simulink library "tetherInternalForces_ul"  (R2018b)
settings: Solver=VariableStepAuto  StartTime=0.0  StopTime=10.0  RelTol=1e-3
values from neighbouring files (symbols this model uses):
  dia_t = 0.01    [tetherInternalForces_ts.m]
  E = 3.8e9    (= 3800000000)    [tetherInternalForces_ts.m]
  mass = 100    [tetherInternalForces_ts.m]
  N = 4    [tetherInternalForces_ts.m]
  zeta = 0.05    [tetherInternalForces_ts.m]
settings Model: Creator=asiddiq2  LastModifiedBy=mcobb

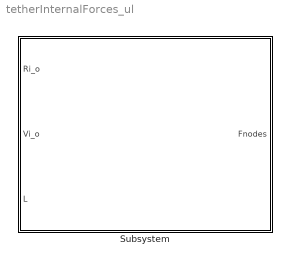
== system tetherInternalForces_ul ==
  Subsystem : Subsystem  mask{N=N, E=E, dia_t=dia_t, mass=mass, zeta=zeta}
      mask prompts: N "Number of nodes (N>=2)"; E "Youngs Modulus (N/m^2)"; dia_t "Tether diameter (m)"; mass "Vehicle Mass (kg)"; zeta "Damping ratio"

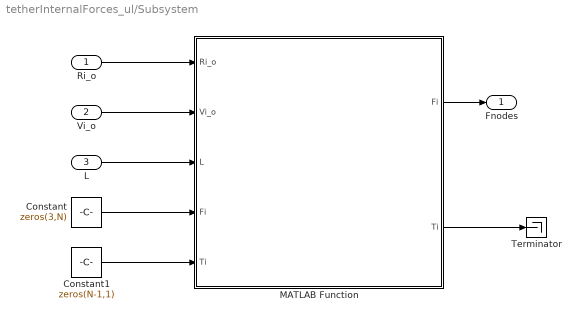
== system tetherInternalForces_ul/Subsystem ==
  Ri_o : Inport
  Vi_o : Inport  Port=2
  L : Inport  Port=3
  Constant : Constant  Value=zeros(3,N)
  Constant1 : Constant  Value=zeros(N-1,1)
  MATLAB Function : MATLAB Function  TreatAsAtomicUnit=on
  Terminator : Terminator
  Fnodes : Outport
  wires:
  Ri_o/1 -> MATLAB Function/1(Ri_o)
  Vi_o/1 -> MATLAB Function/2(Vi_o)
  L/1 -> MATLAB Function/3(L)
  Constant1/1 -> MATLAB Function/5("Ti ")
  MATLAB Function/2(Ti) -> Terminator/1
  MATLAB Function/1(Fi) -> Fnodes/1
  Constant/1 -> MATLAB Function/4("Fi ")

== matlab function tetherInternalForces_ul/Subsystem/MATLAB Function ==
  data: Fi output; Ri_o input; Vi_o input; L input; Fi input; Ti input; N parameter; mass parameter; zeta parameter; dia_t parameter; E parameter; Ti output
 function [Fi,Ti]  = fcn(Ri_o,Vi_o,L,Fi,Ti,N, mass, zeta, dia_t, E)

% cross sectional area
CS = (pi/4)*dia_t^2;

% total spring stiffness
k_tot = E*CS/L;

% total damping coefficient
c_tot = zeta*2*sqrt(k_tot*mass);

% inidividual spring stiffness and damping
k = k_tot*(N-1);
c = c_tot*(N-1);
Li = L/(N-1);

% determine distance between nodes and the derivatives of each element
di = zeros(N-1,1);
direction = zeros(3,N-1);
di_dot = zeros(N-1,1);
Tk = zeros(N-1,1);
Td = zeros(N-1,1);
F_t_i = zeros(3,N);


for ii = 1:N-1
        di(ii) = norm(Ri_o(:,ii+1) - Ri_o(:,ii));
        direction(:,ii) = (Ri_o(:,ii+1) - Ri_o(:,ii))/di(ii);
        di_dot(ii) = dot(Ri_o(:,ii+1) - Ri_o(:,ii),Vi_o(:,ii+1) - Vi_o(:,ii))/di(ii);
    
end

% spring and damper forces
for ii = 1:N-1
    if di(ii) > Li
        Tk(ii) = k*(di(ii) - Li);
        Td(ii) = c*di_dot(ii);
        F_t_i(:,ii) = (Tk(ii) + Td(ii))*direction(:,ii);
        Ti(ii) = norm(F_t_i(:,ii));
    else
        Tk(ii) = 0;
        Td(ii) = 0;
        F_t_i(:,ii) = (Tk(ii) + Td(ii))*direction(:,ii);
        Ti(ii) = norm(F_t_i(:,ii));

    end
end

for ii = 1:N
    if ii == 1
        Fi(:,ii) = F_t_i(:,ii);
    elseif ii > 1 && ii < N
        Fi(:,ii) = F_t_i(:,ii) - F_t_i(:,ii-1);
    elseif ii == N
        Fi(:,ii) = -F_t_i(:,ii-1);
    end
end


% Mitchells version here (Should be equivalen to almost all of the above)
%  di = sqrt(sum(diff(Ri_o,1,2).^2,1))';
%  direction = diff(Ri_o,1,2)./repmat(di',[N-1 1]);
%  di_dot = sum(direction.*diff(Vi_o,1,2),1)';
%  Tk(di>Li) = k*(di(di>Li) - Li)
%  Td(di>Li) = c*di_dot(di>Li)
%  F_t_i(1:end-1) = repmat((Tk' + Td'),[N-1 1]).*direction


end
